simulink model "S_Func_Test"  (R2024b)
settings: Solver=VariableStepAuto  StartTime=0.0  StopTime=10.0  RelTol=1e-3
settings Model: Creator=Gautham  LastModifiedBy=Gautham

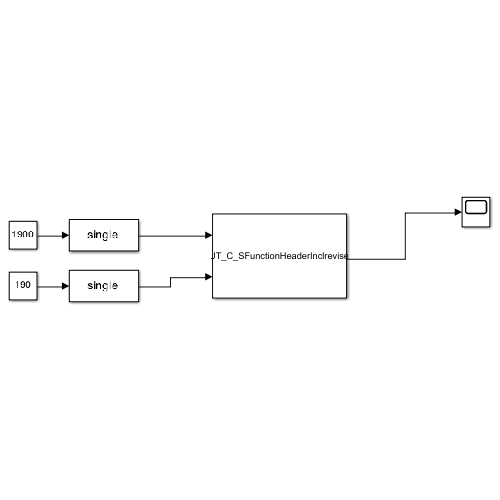
[thumbnail: Simulink's stored preview of the top-level diagram]
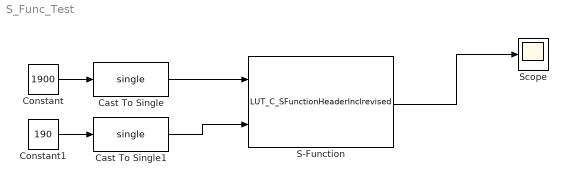
== system S_Func_Test ==
  Cast To Single : DataTypeConversion  OutDataTypeStr=single  SaturateOnIntegerOverflow=off  RndMeth=Floor
  Cast To Single1 : DataTypeConversion  OutDataTypeStr=single  SaturateOnIntegerOverflow=off  RndMeth=Floor
  Constant : Constant  Value=1900
  Constant1 : Constant  Value=190
  S-Function : S-Function  FunctionName=LUT_C_SFunctionHeaderInclrevised  SFunctionDeploymentMode=off  EnableBusSupport=off
  Scope : Scope
  wires:
  Cast To Single/1 -> S-Function/1
  Cast To Single1/1 -> S-Function/2
  Constant/1 -> Cast To Single/1
  Constant1/1 -> Cast To Single1/1
  S-Function/1 -> Scope/1
